simulink model "BMS_ClosedLoop_Harness_Dashboard"  (R2020a)
settings: configuration reference "BMS_Sw_CodeGenConfig" (kept outside this file)
undefined symbols (not defined in the file): Ns_Module, NumModules, SRE
libraries: simulink x2
settings Model: DataDictionary=Battery_System_DD.sldd  EnableAccessToBaseWorkspace=off  Creator=falderis  LastModifiedBy=RolandoA
settings ConfigSetRef: SourceName=BMS_Sw_CodeGenConfig

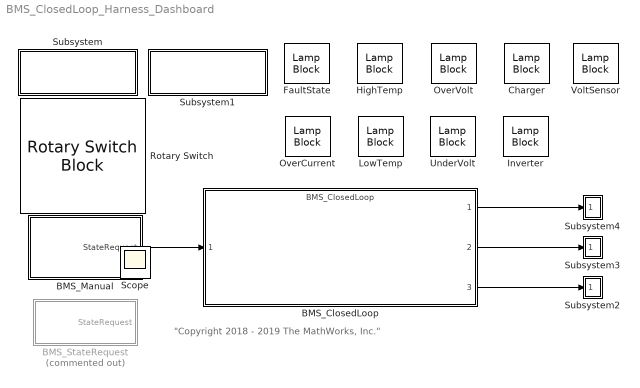
== system BMS_ClosedLoop_Harness_Dashboard ==
  note: "Copyright 2018 - 2019 The MathWorks, Inc."
  BMS_ClosedLoop : ModelReference  ModelNameDialog=BMS_ClosedLoop  SimulationMode=Normal  ModelReferenceVersion=1.550
  BMS_Manual : Subsystem  VariantControl=ManualVariant
  BMS_StateRequest : Subsystem  Commented=on  Variant=on  VariantControlMode=Label  LabelModeActiveChoice=TestSequenceVariant  PropagateVariantConditions=on
  Charger : LampBlock
  FaultState : LampBlock
  HighTemp : LampBlock
  Inverter : LampBlock
  LowTemp : LampBlock
  OverCurrent : LampBlock
  OverVolt : LampBlock
  Rotary Switch : RotarySwitchBlock  LabelPosition=Hide
      settings: Values={{'Bal', 'Chrg', 'Drv'}, [0 1 2]}
  Subsystem : Subsystem  mask(State Request){testCaseChoice=1}
      mask prompts: testCaseChoice "Choose Test Case"
      mask help: Test Sequence Variant
      mask TypeOptions testCaseChoice: 1 | 2 | 3
      mask Callback testCaseChoice:
      | set_param([gcs '/BMS_StateRequest'],'OverrideUsingVariant','TestSequenceVariant');
      | SharedDictionaryObj = Simulink.data.dictionary.open('Shared_DD.sldd');
      | dDataSectObj = getSection(SharedDictionaryObj,'Design Data');
      | TestCase_Variant = find(dDataSectObj,'Name','TestCase');
      | setValue(TestCase_Variant,str2double(get_param(gcb,'testCaseChoice')))
      | 
      | %set_param([gcs '/BMS_StateRequest'],'OverrideUsingVariant','TestSequenceVariant');
      | %assignin('base','TestCase',str2double(get_param(gcb,'testCaseChoice')))
      mask Display: disp('Test Sequence Variant')
  Subsystem1 : Subsystem
      settings: OpenFcn=set_param([gcs '/BMS_StateRequest'],'OverrideUsingVariant','ManualVariant');
      mask Display: disp('Manual Variant')
  Subsystem2 : Subsystem
  Subsystem3 : Subsystem
  Subsystem4 : Subsystem
  UnderVolt : LampBlock
  VoltSensor : LampBlock
  Scope : Scope
  wires:
  BMS_ClosedLoop/2 -> Subsystem3/1(In1)
  BMS_ClosedLoop/3 -> Subsystem2/1(In1)
  BMS_ClosedLoop/1 -> Subsystem4/1(" ")
  BMS_Manual/1(StateRequest) -> BMS_ClosedLoop/1

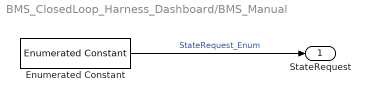
== system BMS_ClosedLoop_Harness_Dashboard/BMS_Manual ==
  Enumerated Constant : simulink/Sources/Enumerated Constant  OutDataTypeStr=Enum: SRE  Value=SRE.Driving  SampleTime=inf
  StateRequest : Outport  VectorParamsAs1DForOutWhenUnconnected=off
  wires:
  Enumerated Constant/1 -> StateRequest/1  "StateRequest_Enum"

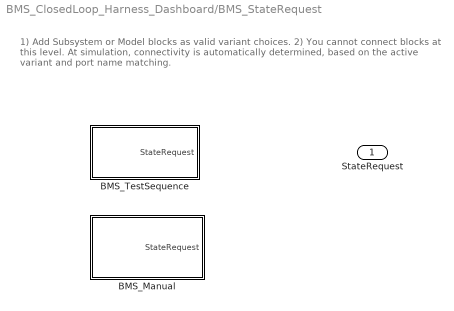
== system BMS_ClosedLoop_Harness_Dashboard/BMS_StateRequest ==
  note: 1) Add Subsystem or Model blocks as valid variant choices.
      | 2) You cannot connect blocks at this level. At simulation, connectivity is automatically
      | determined, based on the active variant and port name matching.
  BMS_Manual : Subsystem  VariantControl=ManualVariant
  BMS_TestSequence : Subsystem  Variant=on  VariantControl=TestSequenceVariant
  StateRequest : Outport  OutDataTypeStr=Enum: SRE  VectorParamsAs1DForOutWhenUnconnected=off

== system BMS_ClosedLoop_Harness_Dashboard/Subsystem ==

== system BMS_ClosedLoop_Harness_Dashboard/Subsystem1 ==

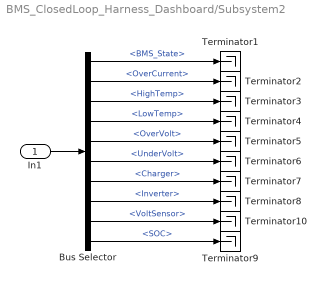
== system BMS_ClosedLoop_Harness_Dashboard/Subsystem2 ==
  In1 : Inport
  Bus Selector : BusSelector  OutputSignals=BMS_State,Faults.OverCurrent,Faults.HighTemp,Faults.LowTemp,Faults.OverVolt,Faults.UnderVolt,Faults.Charger,Faults.Inverter,Faults.VoltSensor,SOC
  Terminator{1..10} (10 alike) : Terminator
  wires:
  Bus Selector/6 -> Terminator6/1  "<UnderVolt>"
  In1/1 -> Bus Selector/1
  Bus Selector/1 -> Terminator1/1  "<BMS_State>"
  Bus Selector/7 -> Terminator7/1  "<Charger>"
  Bus Selector/5 -> Terminator5/1  "<OverVolt>"
  Bus Selector/2 -> Terminator2/1  "<OverCurrent>"
  Bus Selector/3 -> Terminator3/1  "<HighTemp>"
  Bus Selector/4 -> Terminator4/1  "<LowTemp>"
  Bus Selector/8 -> Terminator8/1  "<Inverter>"
  Bus Selector/10 -> Terminator9/1  "<SOC>"
  Bus Selector/9 -> Terminator10/1  "<VoltSensor>"

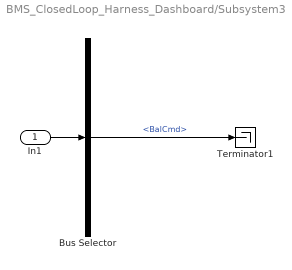
== system BMS_ClosedLoop_Harness_Dashboard/Subsystem3 ==
  In1 : Inport
  Bus Selector : BusSelector  OutputSignals=BalCmd
  Terminator1 : Terminator
  wires:
  Bus Selector/1 -> Terminator1/1  "<BalCmd>"
  In1/1 -> Bus Selector/1

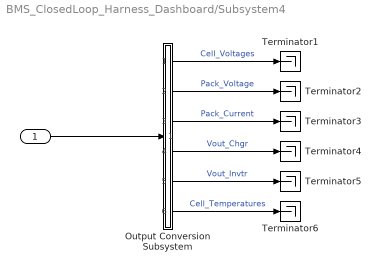
== system BMS_ClosedLoop_Harness_Dashboard/Subsystem4 ==
  " " : Inport
  Output Conversion Subsystem : Subsystem  Tag=__SLT_OCS__  Description=|
      | Signal spec.
      | and routing
      settings: AttributesFormatString=%<Description>
  Terminator{1..6} (6 alike) : Terminator
  wires:
  Output Conversion Subsystem/3(Outport_3) -> Terminator3/1  "Pack_Current"
  Output Conversion Subsystem/1(Outport_1) -> Terminator1/1  "Cell_Voltages"
  " "/1 -> Output Conversion Subsystem/1(Inport_1)
  Output Conversion Subsystem/2(Outport_2) -> Terminator2/1  "Pack_Voltage"
  Output Conversion Subsystem/4(Outport_4) -> Terminator4/1  "Vout_Chgr"
  Output Conversion Subsystem/6(Outport_6) -> Terminator6/1  "Cell_Temperatures"
  Output Conversion Subsystem/5(Outport_5) -> Terminator5/1  "Vout_Invtr"

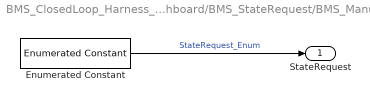
== system BMS_ClosedLoop_Harness_Dashboard/BMS_StateRequest/BMS_Manual ==
  Enumerated Constant : simulink/Sources/Enumerated Constant  OutDataTypeStr=Enum: SRE  Value=SRE(2)  SampleTime=inf
  StateRequest : Outport  VectorParamsAs1DForOutWhenUnconnected=off
  wires:
  Enumerated Constant/1 -> StateRequest/1  "StateRequest_Enum"

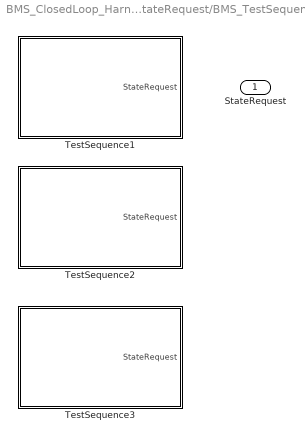
== system BMS_ClosedLoop_Harness_Dashboard/BMS_StateRequest/BMS_TestSequence ==
  TestSequence1 : Test Sequence  TreatAsAtomicUnit=on  VariantControl=TestCase == 1
  TestSequence2 : Test Sequence  TreatAsAtomicUnit=on  VariantControl=TestCase == 2
  TestSequence3 : Test Sequence  TreatAsAtomicUnit=on  VariantControl=TestCase == 3
  " StateRequest" : Outport  VectorParamsAs1DForOutWhenUnconnected=off

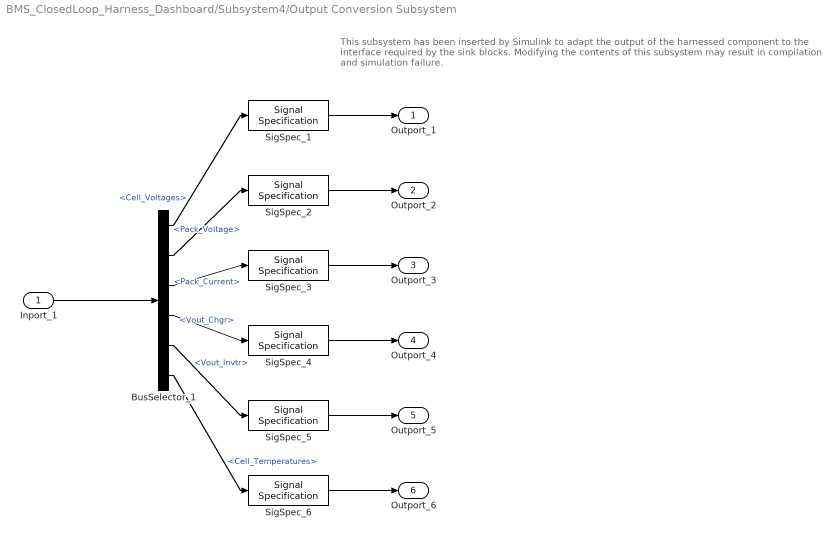
== system BMS_ClosedLoop_Harness_Dashboard/Subsystem4/Output Conversion Subsystem ==
  note: This subsystem has been inserted by Simulink to adapt the output of the harnessed component to the interface required by the sink blocks.
      |  Modifying the contents of this subsystem may result in compilation and simulation failure.
  Inport_1 : Inport
  BusSelector_1 : BusSelector  OutputSignals=Cell_Voltages,Pack_Voltage,Pack_Current,Vout_Chgr,Vout_Invtr,Cell_Temperatures
  SigSpec_1 : SignalSpecification  OutDataTypeStr=single  Dimensions=[Ns_Module*NumModules]
  SigSpec_{2..5} (4 alike) : SignalSpecification  OutDataTypeStr=single  Dimensions=[1]
  SigSpec_6 : SignalSpecification  OutDataTypeStr=single  Dimensions=[Ns_Module*NumModules - 6]
  Outport_1 : Outport  VectorParamsAs1DForOutWhenUnconnected=off
  Outport_2 : Outport  Port=2  VectorParamsAs1DForOutWhenUnconnected=off
  Outport_3 : Outport  Port=3  VectorParamsAs1DForOutWhenUnconnected=off
  Outport_4 : Outport  Port=4  VectorParamsAs1DForOutWhenUnconnected=off
  Outport_5 : Outport  Port=5  VectorParamsAs1DForOutWhenUnconnected=off
  Outport_6 : Outport  Port=6  VectorParamsAs1DForOutWhenUnconnected=off
  wires:
  Inport_1/1 -> BusSelector_1/1
  BusSelector_1/1 -> SigSpec_1/1  "<Cell_Voltages>"
  SigSpec_1/1 -> Outport_1/1
  BusSelector_1/2 -> SigSpec_2/1  "<Pack_Voltage>"
  SigSpec_2/1 -> Outport_2/1
  BusSelector_1/3 -> SigSpec_3/1  "<Pack_Current>"
  SigSpec_3/1 -> Outport_3/1
  BusSelector_1/4 -> SigSpec_4/1  "<Vout_Chgr>"
  SigSpec_4/1 -> Outport_4/1
  BusSelector_1/5 -> SigSpec_5/1  "<Vout_Invtr>"
  SigSpec_5/1 -> Outport_5/1
  BusSelector_1/6 -> SigSpec_6/1  "<Cell_Temperatures>"
  SigSpec_6/1 -> Outport_6/1

== stateflow chart BMS_ClosedLoop_Harness_Dashboard/BMS_StateRequest/BMS_TestSequence/TestSequence1 ==
  settings: stateMachineType=SIMPLIFIED_MACHINE
  state Driving
    StateRequest = SRE.Driving;
  state Balancing
    StateRequest = SRE.Balancing;
  state ChargingAndBalancing
    StateRequest = SRE.Charging;
  state PostChargeBalancing
    StateRequest = SRE.Balancing;
  (default) -> Driving
  Driving -> Balancing : [after(3000,sec)
      | ]
  Balancing -> ChargingAndBalancing : [
      | after(1000,sec)
      | ]
  ChargingAndBalancing -> PostChargeBalancing : [
      | after(5000,sec)
      | ]
  data: StateRequest output Enum: SRE

== stateflow chart BMS_ClosedLoop_Harness_Dashboard/BMS_StateRequest/BMS_TestSequence/TestSequence2 ==
  settings: stateMachineType=SIMPLIFIED_MACHINE
  state Driving
    StateRequest = SRE.Driving;
  state Charging
    StateRequest = SRE.Charging;
  (default) -> Driving
  Driving -> Charging : [after(10000,sec)
      | ]
  data: StateRequest output Enum: SRE

== stateflow chart BMS_ClosedLoop_Harness_Dashboard/BMS_StateRequest/BMS_TestSequence/TestSequence3 ==
  settings: stateMachineType=SIMPLIFIED_MACHINE
  state Charging
    StateRequest = SRE.Charging;
  (default) -> Charging
  data: StateRequest output Enum: SRE
